simulink model "FMC_TopLevel_Fluids"  (R2025a)
settings: Solver=daessc  StartTime=0.0  StopTime=stopTime  RelTol=1e-3
libraries: nesl_utility x1
settings Model: Creator=mu22504  LastModifiedBy=Adam
settings DataIOCC: InspectSignalLogs=on
settings ModelReferenceCC: UseModelRefSolver=on
settings SimscapeCC: SimscapeLogSimulationStatistics=on  SimscapeLogToSDI=on

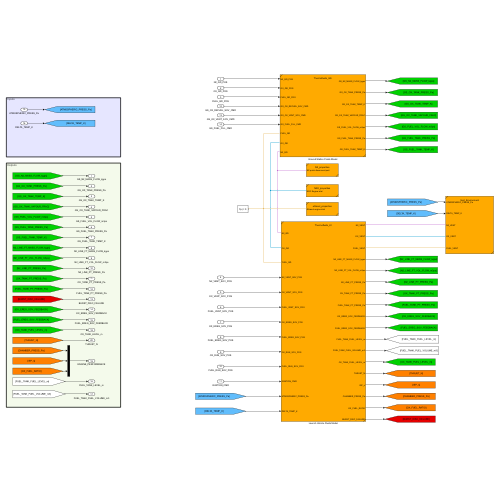
[thumbnail: Simulink's stored preview of the top-level diagram]
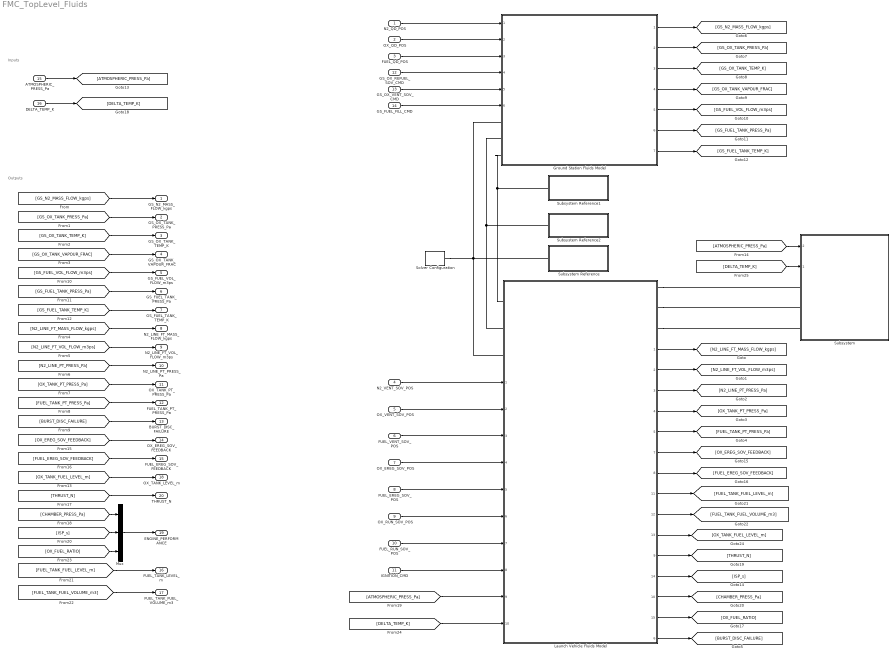
== system FMC_TopLevel_Fluids ==
  note: Inputs
  note: Outputs
  N2_QD_POS : Inport
  OX_QD_POS : Inport  Port=2
  FUEL_QD_POS : Inport  Port=3
  N2_VENT_SOV_POS : Inport  Port=4
  OX_VENT_SOV_POS : Inport  Port=5
  FUEL_VENT_SOV_POS : Inport  Port=6
  OX_EREG_SOV_POS : Inport  Port=7
  FUEL_EREG_SOV_POS : Inport  Port=8
  OX_RUN_SOV_POS : Inport  Port=9
  FUEL_RUN_SOV_POS : Inport  Port=10
  IGNITION_CMD : Inport  Port=11
  GS_OX_REFUEL_SOV_CMD : Inport  Port=12
  GS_OX_VENT_SOV_CMD : Inport  Port=13
  GS_FUEL_FILL_CMD : Inport  Port=14
  ATMOSPHERIC_PRESS_Pa : Inport  Port=15
  DELTA_TEMP_K : Inport  Port=16
  Ground Station Fluids Model : Subsystem  ReferencedSubsystem=Thermofluids_GS
      settings: PortSchema="{\"entries\":[{\"content\":{\"sides\":[{\"content\":{\"connectorIds\":[\"In1\",\"In2\",\"In3\",\"In4\",\"In5\",\"In6\",\"LConn3\",\"LConn2\",\"LConn1\"]},\"type\":\"ConnectorPlacement.EquallySpacedRectSide\",\"uuid\":\"1f0e9dc9-066f-4740-a01f-c871041edae1\"},{\"content\":{\"connectorIds\":[\"Out1\",\"Out2\",\"Out3\",\"Out4\",\"Out5\",\"Out6\",\"Out7\"],\"side\":\"RIGHT\"},\"type\":\"ConnectorPlacement.EquallySpacedRectSide\",\"uuid\":\"23696615-9e6b-4b01-bf34-3e6084e0acc4\"},{\"content\":{\"side\":\"TOP\"},\"type\":\"ConnectorPlacement.EquallySpacedRectSide\",\"uuid\":\"47968613-aa29-4234-9156-172438f99733\"}]},\"type\":\"ConnectorPlacement.EquallySpacedConnector\",\"uuid\":\"3d468e28-1aed-4784-9850-3053ce02f939\"}],\"packageUris\":[\"http://schema.mathworks.com/mf0/Connector/R2020b\"],\"version\":\"1.0\"}"
  Launch Vehicle Fluids Model : Subsystem  ReferencedSubsystem=Thermofluids_LV
      settings: PortSchema="{\"entries\":[{\"content\":{\"sides\":[{\"content\":{\"connectorIds\":[\"LConn1\",\"LConn2\",\"LConn6\",\"In1\",\"In2\",\"In3\",\"In4\",\"In5\",\"In6\",\"In7\",\"In8\",\"In9\",\"In10\"]},\"type\":\"ConnectorPlacement.EquallySpacedRectSide\",\"uuid\":\"a87b0425-c6b8-4d08-a1a8-b3acad5c334a\"},{\"content\":{\"connectorIds\":[\"LConn3\",\"LConn4\",\"LConn5\",\"Out1\",\"Out2\",\"Out3\",\"Out4\",\"Out5\",\"Out7\",\"Out8\",\"Out11\",\"Out12\",\"Out13\",\"Out9\",\"Out14\",\"Out10\",\"Out15\",\"Out6\"],\"side\":\"RIGHT\"},\"type\":\"ConnectorPlacement.EquallySpacedRectSide\",\"uuid\":\"260d6155-6d20-4ed3-9052-698506ea1559\"},{\"content\":{\"side\":\"TOP\"},\"type\":\"ConnectorPlacement.EquallySpacedRectSide\",\"uuid\":\"d266d02d-922b-4f41-b529-513bc445e931\"}]},\"type\":\"ConnectorPlacement.EquallySpacedConnector\",\"uuid\":\"36f51c95-b9e3-4232-bda9-d5a6ea8a2ffc\"}],\"packageUris\":[\"http://schema.mathworks.com/mf0/Connector/R2020b\"],\"version\":\"1.0\"}"
  Mux : Mux  Inputs=3
  Solver Configuration : nesl_utility/Solver Configuration  PhysicalDomain=network_engine_domain  SubClassName=solver  LeftPortType=input  RightPortType=generic  Tones=[]  Harmonics=[]  SimulateNoise=off  Profile=off  UseLocalSampling=off  EnableSwitchedLinearOptims=on  FrequencyDomain=off  UseCCode=off  RelTol=0.001  AbsTol=0.001  MinStep=1e-09  ToWorkspace=off  RevertToSquareIcSolve=off  NumHomotopyIterations=100  PhasorMode=off  PhasorModeNumHarmonics=1  ConsistencySolver=NEWTON_XTOL_AFTER_FTOL  IndexReductionMethod=DerivativeReplacement  DoDC=off  ResidualTolerance=1e-09  ConsistencyTolSource=GLOBAL  ConsistencyAbsTol=0.001  ConsistencyRelTol=0.001  ConsistencyTolFactor=0.001  UseLocalSolver=off  LocalSolverChoice=NE_BACKWARD_EULER_ADVANCER  ResolveIndetEquations=on  FunctionEvalNumThread=1  LocalSolverSampleTime=0.001  DoFixedCost=off  MaxNonlinIter=3  MaxModeIter=2  ComputeImpulses=off  ImpulseIterations=2  LinearAlgebra=auto  LinearAlgebraNumThread=0  EquationFormulation=NE_TIME_EF  DelaysMemoryBudget=1024  AutomaticFiltering=on  FilteringTimeConstant=0.001  PartitionStorageMethod=AS_NEEDED  PartitionMemoryBudget=1024  PartitionMethod=ROBUST  MultibodyUseLocalSolver=off  MultibodyLocalSolverChoice=ODE1  MultibodyLocalSolverSampleTime=0.001
  Subsystem : Subsystem  ReferencedSubsystem=Vent_Environment
      settings: PortSchema="{\"entries\":[{\"content\":{\"sides\":[{\"content\":{\"connectorIds\":[\"In2\",\"In1\",\"LConn1\",\"LConn2\",\"LConn3\"]},\"type\":\"ConnectorPlacement.EquallySpacedRectSide\",\"uuid\":\"bd7d0a07-10d0-4924-b95d-a248e6f85938\"},{\"content\":{\"side\":\"RIGHT\"},\"type\":\"ConnectorPlacement.EquallySpacedRectSide\",\"uuid\":\"b3422b98-d44b-49ab-81f4-e36fa4aede12\"},{\"content\":{\"side\":\"TOP\"},\"type\":\"ConnectorPlacement.EquallySpacedRectSide\",\"uuid\":\"1874bb35-0acd-4282-addc-685d743a7a07\"}]},\"type\":\"ConnectorPlacement.EquallySpacedConnector\",\"uuid\":\"9c27831b-ff3d-4fc6-a9f6-eb8523648c1b\"}],\"packageUris\":[\"http://schema.mathworks.com/mf0/Connector/R2020b\"],\"version\":\"1.0\"}"
  Subsystem Reference : Subsystem  ReferencedSubsystem=ethanol_properties
  Subsystem Reference1 : Subsystem  ReferencedSubsystem=N2_properties
  Subsystem Reference2 : Subsystem  ReferencedSubsystem=N2O_properties
  GS_N2_MASS_FLOW_kgps : Outport
  GS_OX_TANK_PRESS_Pa : Outport  Port=2
  GS_OX_TANK_TEMP_K : Outport  Port=3
  GS_OX_TANK_VAPOUR_FRAC : Outport  Port=4
  GS_FUEL_VOL_FLOW_m3ps : Outport  Port=5
  GS_FUEL_TANK_PRESS_Pa : Outport  Port=6
  GS_FUEL_TANK_TEMP_K : Outport  Port=7
  N2_LINE_FT_MASS_FLOW_kgps : Outport  Port=8
  N2_LINE_FT_VOL_FLOW_m3ps : Outport  Port=9
  N2_LINE_PT_PRESS_Pa : Outport  Port=10
  OX_TANK_PT_PRESS_Pa : Outport  Port=11
  FUEL_TANK_PT_PRESS_Pa : Outport  Port=12
  BURST_DISC_FAILURE : Outport  Port=13
  OX_EREG_SOV_FEEDBACK : Outport  Port=14
  FUEL_EREG_SOV_FEEDBACK : Outport  Port=15
  FUEL_TANK_LEVEL_m : Outport  Port=16
  FUEL_TANK_FUEL_VOLUME_m3 : Outport  Port=17
  OX_TANK_LEVEL_m : Outport  Port=18
  ENGINE_PERFORMANCE : Outport  Port=19
  THRUST_N : Outport  Port=20
  wires:
  Launch Vehicle Fluids Model/1 -> [N2_LINE_FT_MASS_FLOW_kgps]
  Launch Vehicle Fluids Model/2 -> [N2_LINE_FT_VOL_FLOW_m3ps]
  Launch Vehicle Fluids Model/3 -> [N2_LINE_PT_PRESS_Pa]
  Launch Vehicle Fluids Model/4 -> [OX_TANK_PT_PRESS_Pa]
  Launch Vehicle Fluids Model/5 -> [FUEL_TANK_PT_PRESS_Pa]
  Launch Vehicle Fluids Model/6 -> [BURST_DISC_FAILURE]
  Ground Station Fluids Model/1 -> [GS_N2_MASS_FLOW_kgps]
  Ground Station Fluids Model/2 -> [GS_OX_TANK_PRESS_Pa]
  Ground Station Fluids Model/3 -> [GS_OX_TANK_TEMP_K]
  Ground Station Fluids Model/4 -> [GS_OX_TANK_VAPOUR_FRAC]
  [GS_N2_MASS_FLOW_kgps] -> GS_N2_MASS_FLOW_kgps/1
  [GS_OX_TANK_PRESS_Pa] -> GS_OX_TANK_PRESS_Pa/1
  [GS_OX_TANK_TEMP_K] -> GS_OX_TANK_TEMP_K/1
  [GS_OX_TANK_VAPOUR_FRAC] -> GS_OX_TANK_VAPOUR_FRAC/1
  [N2_LINE_FT_MASS_FLOW_kgps] -> N2_LINE_FT_MASS_FLOW_kgps/1
  [BURST_DISC_FAILURE] -> BURST_DISC_FAILURE/1
  [FUEL_TANK_PT_PRESS_Pa] -> FUEL_TANK_PT_PRESS_Pa/1
  [OX_TANK_PT_PRESS_Pa] -> OX_TANK_PT_PRESS_Pa/1
  [N2_LINE_PT_PRESS_Pa] -> N2_LINE_PT_PRESS_Pa/1
  [N2_LINE_FT_VOL_FLOW_m3ps] -> N2_LINE_FT_VOL_FLOW_m3ps/1
  Ground Station Fluids Model/5 -> [GS_FUEL_VOL_FLOW_m3ps]
  Ground Station Fluids Model/6 -> [GS_FUEL_TANK_PRESS_Pa]
  Ground Station Fluids Model/7 -> [GS_FUEL_TANK_TEMP_K]
  [GS_FUEL_VOL_FLOW_m3ps] -> GS_FUEL_VOL_FLOW_m3ps/1
  [GS_FUEL_TANK_PRESS_Pa] -> GS_FUEL_TANK_PRESS_Pa/1
  [GS_FUEL_TANK_TEMP_K] -> GS_FUEL_TANK_TEMP_K/1
  [DELTA_TEMP_K] -> Subsystem/1
  [ATMOSPHERIC_PRESS_Pa] -> Subsystem/2
  Launch Vehicle Fluids Model/7 -> [OX_EREG_SOV_FEEDBACK]
  Launch Vehicle Fluids Model/8 -> [FUEL_EREG_SOV_FEEDBACK]
  [OX_EREG_SOV_FEEDBACK] -> OX_EREG_SOV_FEEDBACK/1
  [FUEL_EREG_SOV_FEEDBACK] -> FUEL_EREG_SOV_FEEDBACK/1
  Launch Vehicle Fluids Model/9 -> [THRUST_N]
  Launch Vehicle Fluids Model/10 -> [CHAMBER_PRESS_Pa]
  Launch Vehicle Fluids Model/12 -> [FUEL_TANK_FUEL_VOLUME_m3]
  Launch Vehicle Fluids Model/11 -> [FUEL_TANK_FUEL_LEVEL_m]
  [FUEL_TANK_FUEL_VOLUME_m3] -> FUEL_TANK_FUEL_VOLUME_m3/1
  [FUEL_TANK_FUEL_LEVEL_m] -> FUEL_TANK_LEVEL_m/1
  N2_QD_POS/1 -> Ground Station Fluids Model/1
  OX_QD_POS/1 -> Ground Station Fluids Model/2
  N2_VENT_SOV_POS/1 -> Launch Vehicle Fluids Model/1
  OX_VENT_SOV_POS/1 -> Launch Vehicle Fluids Model/2
  FUEL_VENT_SOV_POS/1 -> Launch Vehicle Fluids Model/3
  OX_EREG_SOV_POS/1 -> Launch Vehicle Fluids Model/4
  FUEL_EREG_SOV_POS/1 -> Launch Vehicle Fluids Model/5
  OX_RUN_SOV_POS/1 -> Launch Vehicle Fluids Model/6
  FUEL_RUN_SOV_POS/1 -> Launch Vehicle Fluids Model/7
  IGNITION_CMD/1 -> Launch Vehicle Fluids Model/8
  Launch Vehicle Fluids Model/13 -> [OX_TANK_FUEL_LEVEL_m]
  [OX_TANK_FUEL_LEVEL_m] -> OX_TANK_LEVEL_m/1
  FUEL_QD_POS/1 -> Ground Station Fluids Model/3
  GS_OX_REFUEL_SOV_CMD/1 -> Ground Station Fluids Model/4
  GS_OX_VENT_SOV_CMD/1 -> Ground Station Fluids Model/5
  GS_FUEL_FILL_CMD/1 -> Ground Station Fluids Model/6
  ATMOSPHERIC_PRESS_Pa/1 -> [ATMOSPHERIC_PRESS_Pa]
  Launch Vehicle Fluids Model/14 -> [ISP_s]
  Launch Vehicle Fluids Model/15 -> [OX_FUEL_RATIO]
  [OX_FUEL_RATIO] -> Mux/3
  DELTA_TEMP_K/1 -> [DELTA_TEMP_K]
  [ATMOSPHERIC_PRESS_Pa] -> Launch Vehicle Fluids Model/9
  [DELTA_TEMP_K] -> Launch Vehicle Fluids Model/10
  Mux/1 -> ENGINE_PERFORMANCE/1
  [CHAMBER_PRESS_Pa] -> Mux/1
  [ISP_s] -> Mux/2
  [THRUST_N] -> THRUST_N/1
  connections:
  Ground Station Fluids Model/LConn1 -- Subsystem Reference1/LConn1 -- Launch Vehicle Fluids Model/LConn1
  Launch Vehicle Fluids Model/LConn2 -- Subsystem Reference2/LConn1 -- Ground Station Fluids Model/LConn2
  Subsystem Reference/LConn1 -- Ground Station Fluids Model/LConn3 -- Solver Configuration/RConn1 -- Launch Vehicle Fluids Model/LConn6
  Launch Vehicle Fluids Model/LConn3 -- Subsystem/LConn1
  Launch Vehicle Fluids Model/LConn4 -- Subsystem/LConn2
  Launch Vehicle Fluids Model/LConn5 -- Subsystem/LConn3
